simulink model "bicopter_control_comparison"  (R2023a)
settings: Solver=VariableStepAuto  StartTime=0.0  StopTime=20.0  RelTol=1e-3
libraries: fuzblock x4, simulink_extras x1
settings Model: Creator=KIIT  LastModifiedBy=tanay
settings OptimizationCC: ReuseModelBlockBuffer=off
settings DebuggingCC: UnconnectedInputMsg=warning  UnconnectedOutputMsg=warning  UnconnectedLineMsg=warning
settings ModelReferenceCC: EnableRefExpFcnMdlSchedulingChecks=on
settings RTWCC: DLArmComputeVersion=19.05

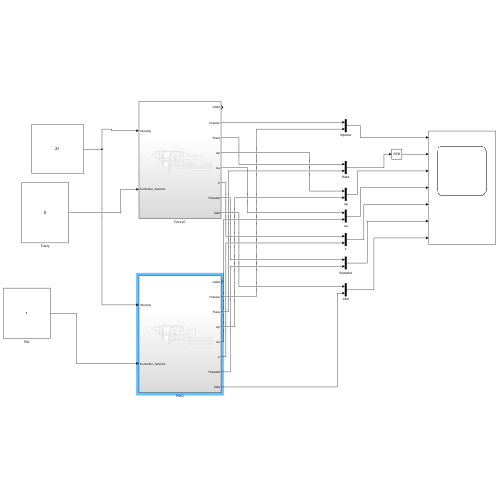
[thumbnail: Simulink's stored preview of the top-level diagram]
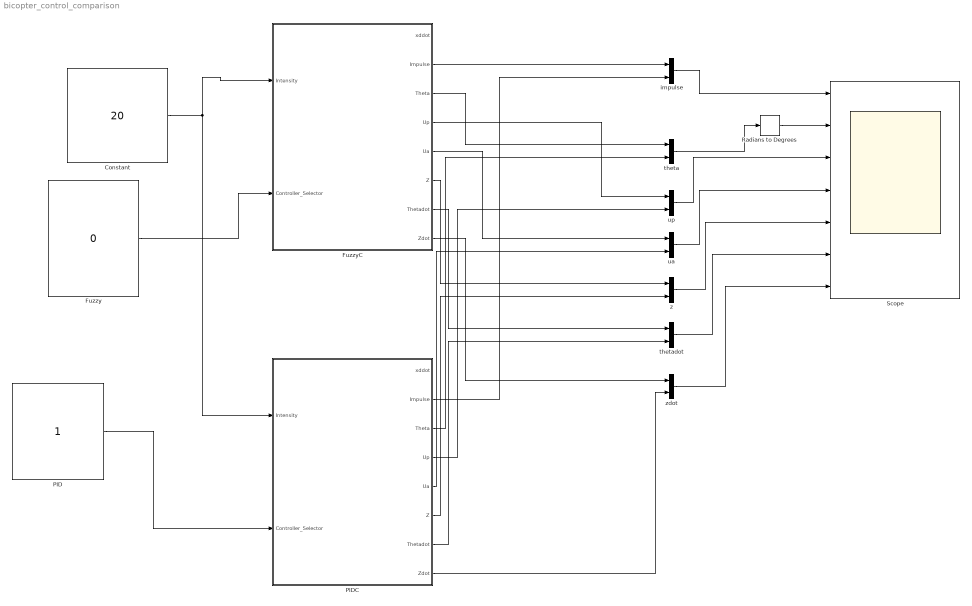
== system bicopter_control_comparison ==
  Constant : Constant  Value=20
  Fuzzy : Constant  Value=0
  FuzzyC : Subsystem
  PID : Constant
  PIDC : Subsystem
  Radians to Degrees : simulink_extras/Transformations/Radians to Degrees
  Scope : Scope  NumInputPorts=7
  impulse : Mux  Inputs=2
  theta : Mux  Inputs=2
  thetadot : Mux  Inputs=2
  ua : Mux  Inputs=2
  up : Mux  Inputs=2
  z : Mux  Inputs=2
  zdot : Mux  Inputs=2
  wires:
  Constant/1 -> FuzzyC/1(Intensity), PIDC/1(Intensity)
  PID/1 -> PIDC/2(Controller_Selector)
  Fuzzy/1 -> FuzzyC/2(Controller_Selector)
  FuzzyC/2(Impulse) -> impulse/1
  PIDC/2(Impulse) -> impulse/2
  FuzzyC/3(Theta) -> theta/1
  PIDC/3(Theta) -> theta/2
  FuzzyC/4(Up) -> up/1
  PIDC/4(Up) -> up/2
  FuzzyC/5(Ua) -> ua/1
  FuzzyC/6(Z) -> z/1
  FuzzyC/7(Thetadot) -> thetadot/1
  FuzzyC/8(Zdot) -> zdot/1
  PIDC/5(Ua) -> ua/2
  PIDC/6(Z) -> z/2
  PIDC/7(Thetadot) -> thetadot/2
  PIDC/8(Zdot) -> zdot/2
  impulse/1 -> Scope/1
  up/1 -> Scope/3
  ua/1 -> Scope/4
  z/1 -> Scope/5
  thetadot/1 -> Scope/6
  zdot/1 -> Scope/7
  theta/1 -> Radians to Degrees/1
  Radians to Degrees/1 -> Scope/2

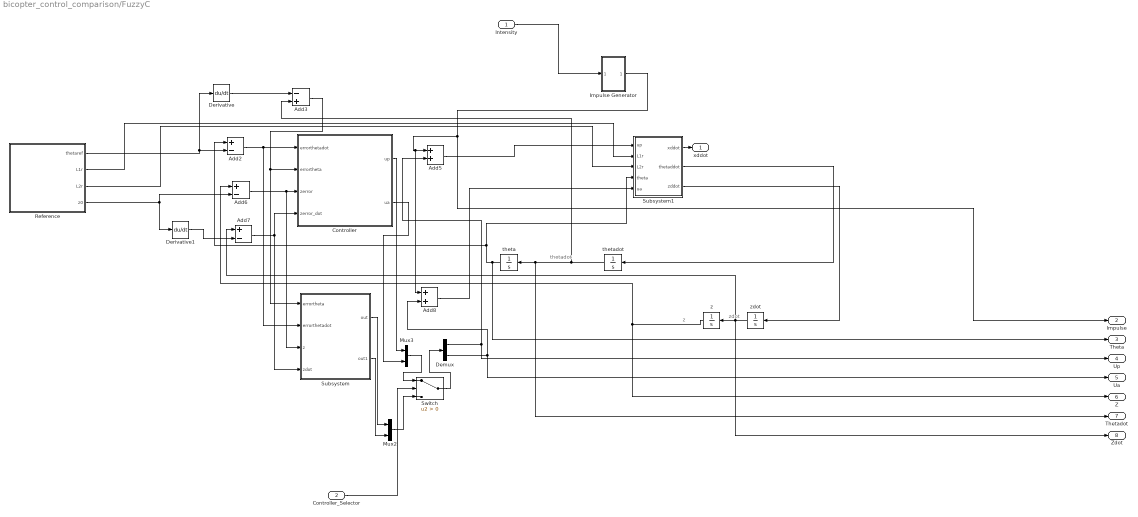
== system bicopter_control_comparison/FuzzyC ==
  note: z
  note: zdot
  note: thetadot
  Intensity : Inport
  Controller_Selector : Inport  Port=2
  Add2 : Sum  Inputs=+-
  Add3 : Sum  Inputs=-+
  Add5 : Sum
  Add6 : Sum  Inputs=+-
  Add7 : Sum  Inputs=+-
  Add8 : Sum
  Controller : Subsystem
  Demux : Demux  Outputs=2
  Derivative : Derivative
  Derivative1 : Derivative
  Impulse Generator : Subsystem
  Mux2 : Mux  Inputs=2
  Mux3 : Mux  Inputs=2
  Reference : MATLAB Function  TreatAsAtomicUnit=on
  Subsystem : Subsystem
  Subsystem1 : Subsystem
  Switch : Switch  Criteria=u2 > Threshold  SaturateOnIntegerOverflow=off  InputSameDT=off
  theta : Integrator  WrapState=on
  thetadot : Integrator
  z : Integrator
  zdot : Integrator
  xddot : Outport
  Impulse : Outport  Port=2
  Theta : Outport  Port=3
  Up : Outport  Port=4
  Ua : Outport  Port=5
  Z : Outport  Port=6
  Thetadot : Outport  Port=7
  Zdot : Outport  Port=8
  wires:
  Add7/1 -> Subsystem/4(zdot), Controller/4(zerror_dot)
  Reference/4(z0) -> Derivative1/1, Add6/2
  Intensity/1 -> Impulse Generator/1(Intensity)
  Subsystem/2(out1) -> Mux2/2
  zdot/1 -> Zdot/1, Add7/1, z/1
  Reference/1(thetaref) -> Add2/2, Derivative/1
  Add6/1 -> Subsystem/3(z), Controller/3(zerror)
  Controller/2(ua) -> Mux3/2
  z/1 -> Z/1, Add6/1
  Add2/1 -> Subsystem/2(errorthetadot), Controller/1(errorthetadot)
  Add3/1 -> Subsystem/1(errortheta), Controller/2(errortheta)
  Add5/1 -> Subsystem1/1(up)
  Subsystem/1(out) -> Mux2/1
  theta/1 -> Theta/1, Subsystem1/4(theta), Add2/1
  Demux/1 -> Add5/2, Up/1
  Derivative/1 -> Add3/1
  Controller/1(up) -> Mux3/1
  Impulse Generator/1(Out1) -> Impulse/1, Add8/1, Add5/1
  Reference/2(L1r) -> Subsystem1/2(L1r)
  Derivative1/1 -> Add7/2
  Subsystem1/3(zddot) -> zdot/1
  Subsystem1/1(xddot) -> xddot/1
  thetadot/1 -> Add3/2, Thetadot/1, theta/1
  Demux/2 -> Add8/2, Ua/1
  Switch/1 -> Demux/1
  Mux2/1 -> Switch/3
  Add8/1 -> Subsystem1/5(ua)
  Mux3/1 -> Switch/1
  Subsystem1/2(thetaddot) -> thetadot/1
  Controller_Selector/1 -> Switch/2
  Reference/3(L2r) -> Subsystem1/3(L2r)

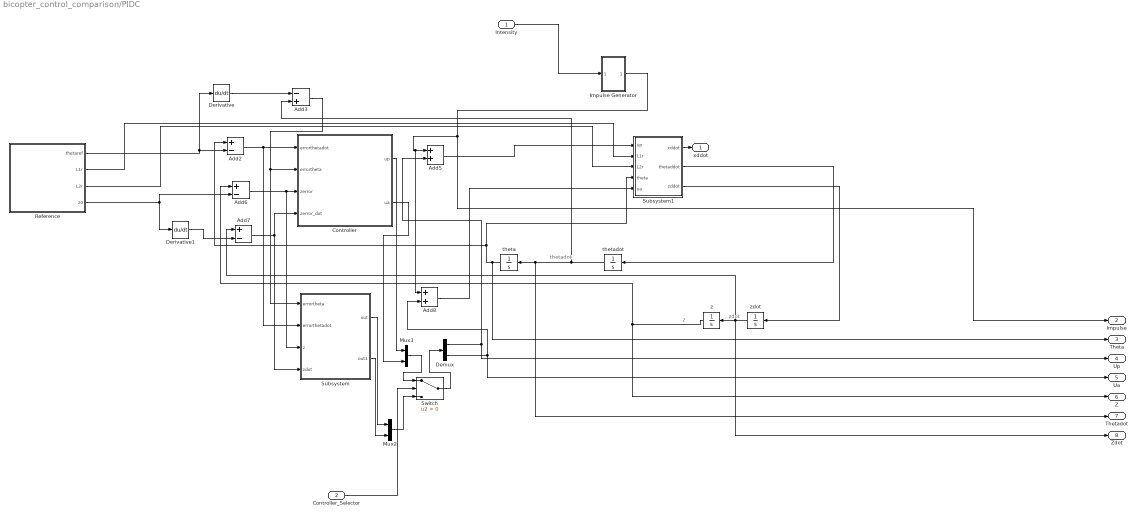
== system bicopter_control_comparison/PIDC ==
  note: z
  note: zdot
  note: thetadot
  Intensity : Inport
  Controller_Selector : Inport  Port=2
  Add2 : Sum  Inputs=+-
  Add3 : Sum  Inputs=-+
  Add5 : Sum
  Add6 : Sum  Inputs=+-
  Add7 : Sum  Inputs=+-
  Add8 : Sum
  Controller : Subsystem
  Demux : Demux  Outputs=2
  Derivative : Derivative
  Derivative1 : Derivative
  Impulse Generator : Subsystem
  Mux2 : Mux  Inputs=2
  Mux3 : Mux  Inputs=2
  Reference : MATLAB Function  TreatAsAtomicUnit=on
  Subsystem : Subsystem
  Subsystem1 : Subsystem
  Switch : Switch  Criteria=u2 > Threshold  SaturateOnIntegerOverflow=off  InputSameDT=off
  theta : Integrator  WrapState=on
  thetadot : Integrator
  z : Integrator
  zdot : Integrator
  xddot : Outport
  Impulse : Outport  Port=2
  Theta : Outport  Port=3
  Up : Outport  Port=4
  Ua : Outport  Port=5
  Z : Outport  Port=6
  Thetadot : Outport  Port=7
  Zdot : Outport  Port=8
  wires:
  Add7/1 -> Subsystem/4(zdot), Controller/4(zerror_dot)
  Reference/4(z0) -> Derivative1/1, Add6/2
  Intensity/1 -> Impulse Generator/1(Intensity)
  Subsystem/2(out1) -> Mux2/2
  zdot/1 -> Zdot/1, Add7/1, z/1
  Reference/1(thetaref) -> Add2/2, Derivative/1
  Add6/1 -> Subsystem/3(z), Controller/3(zerror)
  Controller/2(ua) -> Mux3/2
  z/1 -> Z/1, Add6/1
  Add2/1 -> Subsystem/2(errorthetadot), Controller/1(errorthetadot)
  Add3/1 -> Subsystem/1(errortheta), Controller/2(errortheta)
  Add5/1 -> Subsystem1/1(up)
  Subsystem/1(out) -> Mux2/1
  theta/1 -> Theta/1, Subsystem1/4(theta), Add2/1
  Demux/1 -> Add5/2, Up/1
  Derivative/1 -> Add3/1
  Controller/1(up) -> Mux3/1
  Impulse Generator/1(Out1) -> Impulse/1, Add8/1, Add5/1
  Reference/2(L1r) -> Subsystem1/2(L1r)
  Derivative1/1 -> Add7/2
  Subsystem1/3(zddot) -> zdot/1
  Subsystem1/1(xddot) -> xddot/1
  thetadot/1 -> Add3/2, Thetadot/1, theta/1
  Demux/2 -> Add8/2, Ua/1
  Switch/1 -> Demux/1
  Mux2/1 -> Switch/3
  Add8/1 -> Subsystem1/5(ua)
  Mux3/1 -> Switch/1
  Subsystem1/2(thetaddot) -> thetadot/1
  Controller_Selector/1 -> Switch/2
  Reference/3(L2r) -> Subsystem1/3(L2r)

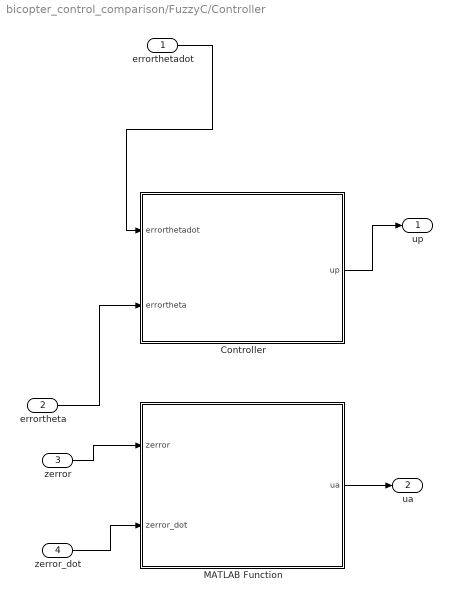
== system bicopter_control_comparison/FuzzyC/Controller ==
  errorthetadot : Inport
  errortheta : Inport  Port=2
  zerror : Inport  Port=3
  zerror_dot : Inport  Port=4
  Controller : MATLAB Function  TreatAsAtomicUnit=on
  MATLAB Function : MATLAB Function  TreatAsAtomicUnit=on
  up : Outport
  ua : Outport  Port=2
  wires:
  errortheta/1 -> Controller/2(errortheta)
  MATLAB Function/1(ua) -> ua/1
  errorthetadot/1 -> Controller/1(errorthetadot)
  zerror/1 -> MATLAB Function/1(zerror)
  Controller/1(up) -> up/1
  zerror_dot/1 -> MATLAB Function/2(zerror_dot)

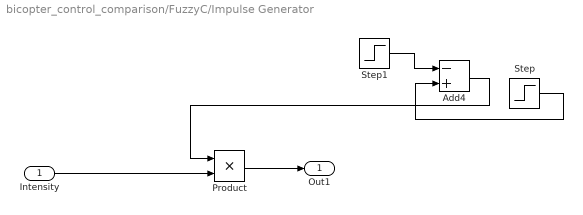
== system bicopter_control_comparison/FuzzyC/Impulse Generator ==
  Intensity : Inport
  Add4 : Sum  Inputs=-+
  Product : Product
  Step : Step  SampleTime=0
  Step1 : Step  Time=2  SampleTime=0
  Out1 : Outport
  wires:
  Step1/1 -> Add4/1
  Step/1 -> Add4/2
  Add4/1 -> Product/1
  Product/1 -> Out1/1
  Intensity/1 -> Product/2

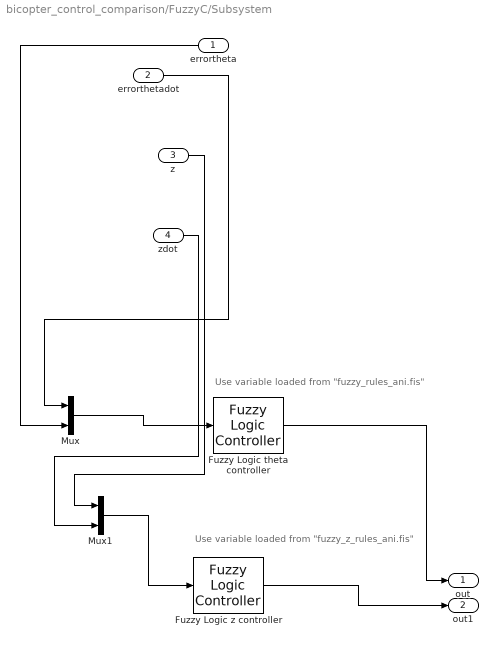
== system bicopter_control_comparison/FuzzyC/Subsystem ==
  note: Use variable loaded from "fuzzy_rules_ani.fis"
  note: Use variable loaded from "fuzzy_z_rules_ani.fis"
  errortheta : Inport
  errorthetadot : Inport  Port=2
  z : Inport  Port=3
  zdot : Inport  Port=4
  Fuzzy Logic theta controller : fuzblock/Fuzzy Logic  Controller  FIS=fuzzy_rules_ani  OutputSampleNumber=101  DataType=double  FuzzifiedInputs=off  RuleFiringStrengths=off  RuleOutputs=off  AggregatedOutputs=off  SimulateUsing=Interpreted execution  OutOfRangeInputValueMessage=warning  NoRuleFiredMessage=warning  EmptyOutputFuzzySetMessage=warning
  Fuzzy Logic z controller : fuzblock/Fuzzy Logic  Controller  FIS=fuzzy_z_rules_ani  OutputSampleNumber=101  DataType=double  FuzzifiedInputs=off  RuleFiringStrengths=off  RuleOutputs=off  AggregatedOutputs=off  SimulateUsing=Interpreted execution  OutOfRangeInputValueMessage=warning  NoRuleFiredMessage=warning  EmptyOutputFuzzySetMessage=warning
  Mux : Mux  Inputs=2
  Mux1 : Mux  Inputs=2
  out : Outport
  out1 : Outport  Port=2
  wires:
  Mux1/1 -> Fuzzy Logic z controller/1
  z/1 -> Mux1/1
  Mux/1 -> Fuzzy Logic theta controller/1
  errorthetadot/1 -> Mux/1
  Fuzzy Logic z controller/1 -> out1/1
  zdot/1 -> Mux1/2
  Fuzzy Logic theta controller/1 -> out/1
  errortheta/1 -> Mux/2

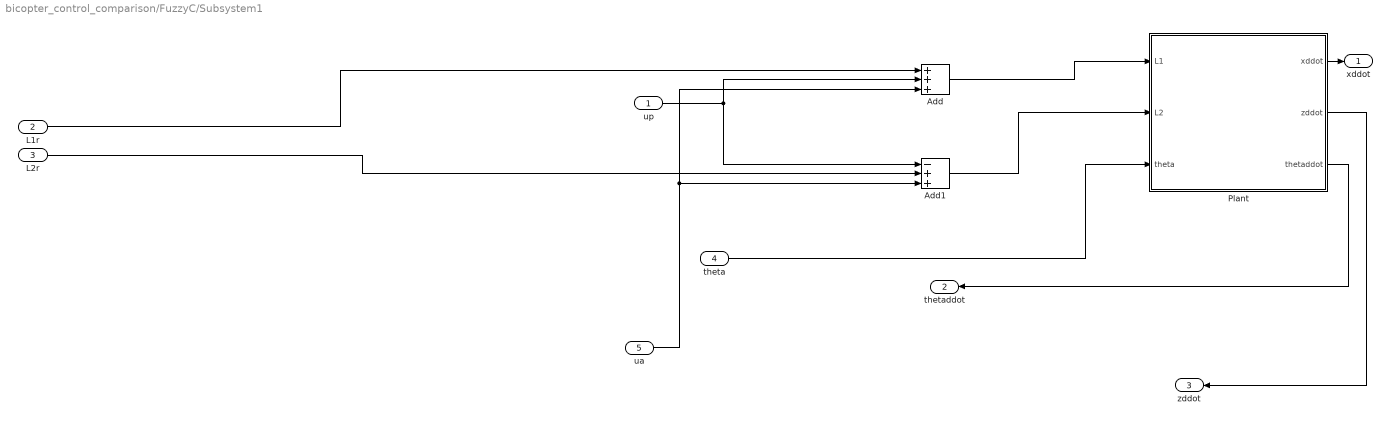
== system bicopter_control_comparison/FuzzyC/Subsystem1 ==
  up : Inport
  L1r : Inport  Port=2
  L2r : Inport  Port=3
  theta : Inport  Port=4
  ua : Inport  Port=5
  Add : Sum  Inputs=+++
  Add1 : Sum  Inputs=-++
  Plant : MATLAB Function  TreatAsAtomicUnit=on
  xddot : Outport
  thetaddot : Outport  Port=2
  zddot : Outport  Port=3
  wires:
  up/1 -> Add/2, Add1/1
  ua/1 -> Add/3, Add1/3
  L1r/1 -> Add/1
  Add1/1 -> Plant/2(L2)
  Plant/1(xddot) -> xddot/1
  Add/1 -> Plant/1(L1)
  L2r/1 -> Add1/2
  theta/1 -> Plant/3(theta)
  Plant/3(thetaddot) -> thetaddot/1
  Plant/2(zddot) -> zddot/1

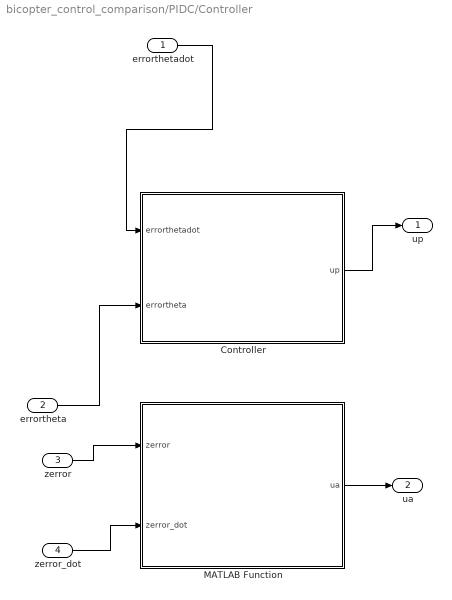
== system bicopter_control_comparison/PIDC/Controller ==
  errorthetadot : Inport
  errortheta : Inport  Port=2
  zerror : Inport  Port=3
  zerror_dot : Inport  Port=4
  Controller : MATLAB Function  TreatAsAtomicUnit=on
  MATLAB Function : MATLAB Function  TreatAsAtomicUnit=on
  up : Outport
  ua : Outport  Port=2
  wires:
  errortheta/1 -> Controller/2(errortheta)
  MATLAB Function/1(ua) -> ua/1
  errorthetadot/1 -> Controller/1(errorthetadot)
  zerror/1 -> MATLAB Function/1(zerror)
  Controller/1(up) -> up/1
  zerror_dot/1 -> MATLAB Function/2(zerror_dot)

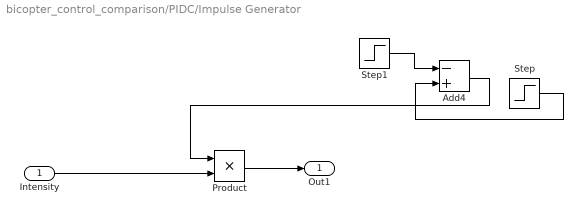
== system bicopter_control_comparison/PIDC/Impulse Generator ==
  Intensity : Inport
  Add4 : Sum  Inputs=-+
  Product : Product
  Step : Step  SampleTime=0
  Step1 : Step  Time=2  SampleTime=0
  Out1 : Outport
  wires:
  Step1/1 -> Add4/1
  Step/1 -> Add4/2
  Add4/1 -> Product/1
  Product/1 -> Out1/1
  Intensity/1 -> Product/2

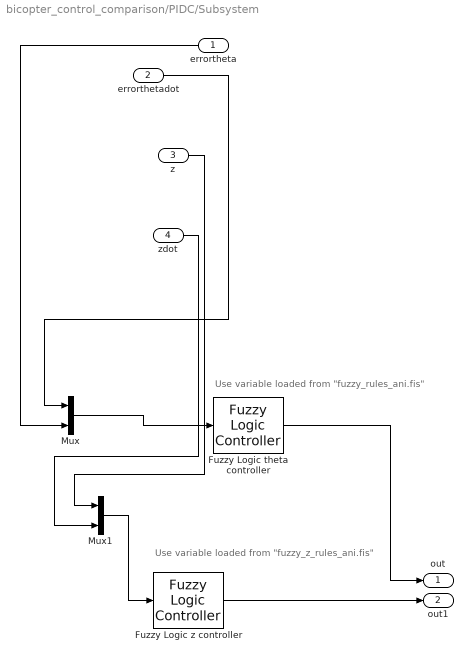
== system bicopter_control_comparison/PIDC/Subsystem ==
  note: Use variable loaded from "fuzzy_rules_ani.fis"
  note: Use variable loaded from "fuzzy_z_rules_ani.fis"
  errortheta : Inport
  errorthetadot : Inport  Port=2
  z : Inport  Port=3
  zdot : Inport  Port=4
  Fuzzy Logic theta controller : fuzblock/Fuzzy Logic  Controller  FIS=fuzzy_rules_ani  OutputSampleNumber=101  DataType=double  FuzzifiedInputs=off  RuleFiringStrengths=off  RuleOutputs=off  AggregatedOutputs=off  SimulateUsing=Interpreted execution  OutOfRangeInputValueMessage=warning  NoRuleFiredMessage=warning  EmptyOutputFuzzySetMessage=warning
  Fuzzy Logic z controller : fuzblock/Fuzzy Logic  Controller  FIS=fuzzy_z_rules_ani  OutputSampleNumber=101  DataType=double  FuzzifiedInputs=off  RuleFiringStrengths=off  RuleOutputs=off  AggregatedOutputs=off  SimulateUsing=Interpreted execution  OutOfRangeInputValueMessage=warning  NoRuleFiredMessage=warning  EmptyOutputFuzzySetMessage=warning
  Mux : Mux  Inputs=2
  Mux1 : Mux  Inputs=2
  out : Outport
  out1 : Outport  Port=2
  wires:
  Mux1/1 -> Fuzzy Logic z controller/1
  z/1 -> Mux1/1
  Mux/1 -> Fuzzy Logic theta controller/1
  errorthetadot/1 -> Mux/1
  Fuzzy Logic z controller/1 -> out1/1
  zdot/1 -> Mux1/2
  Fuzzy Logic theta controller/1 -> out/1
  errortheta/1 -> Mux/2

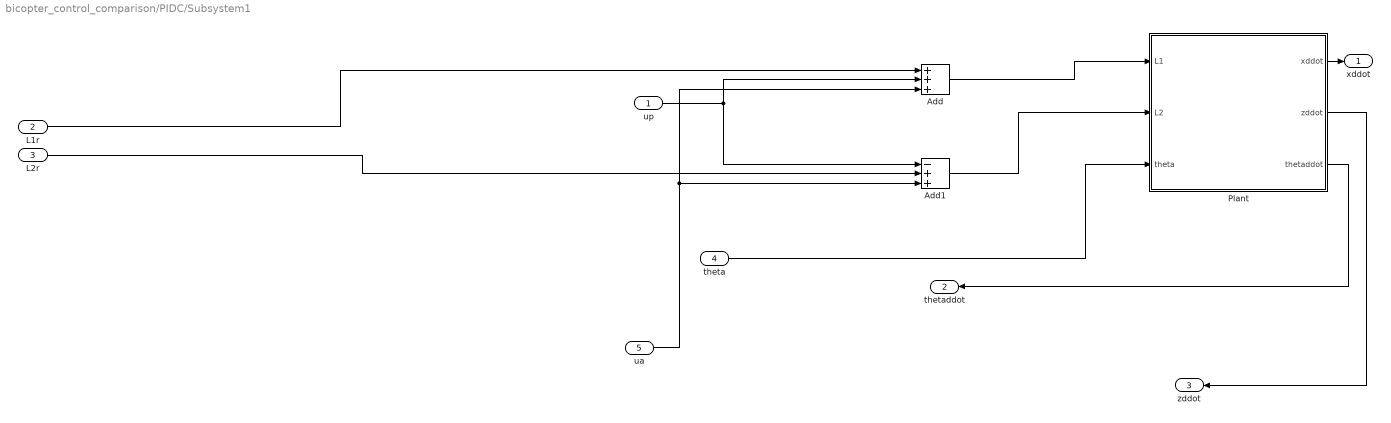
== system bicopter_control_comparison/PIDC/Subsystem1 ==
  up : Inport
  L1r : Inport  Port=2
  L2r : Inport  Port=3
  theta : Inport  Port=4
  ua : Inport  Port=5
  Add : Sum  Inputs=+++
  Add1 : Sum  Inputs=-++
  Plant : MATLAB Function  TreatAsAtomicUnit=on
  xddot : Outport
  thetaddot : Outport  Port=2
  zddot : Outport  Port=3
  wires:
  up/1 -> Add/2, Add1/1
  ua/1 -> Add/3, Add1/3
  L1r/1 -> Add/1
  Add1/1 -> Plant/2(L2)
  Plant/1(xddot) -> xddot/1
  Add/1 -> Plant/1(L1)
  L2r/1 -> Add1/2
  theta/1 -> Plant/3(theta)
  Plant/3(thetaddot) -> thetaddot/1
  Plant/2(zddot) -> zddot/1

== matlab function bicopter_control_comparison/FuzzyC/Subsystem1/Plant ==
  data: L1 input; xddot output; L2 input; theta input; zddot output; thetaddot output
function [xddot, zddot, thetaddot] = fcn(L1, L2, theta)
m = 2;
Iy = 0.2;
g = 9.8;
d = 0.2;
k1 = 24;
k2 = 7;
o1 = -(1/m)*(L1+L2)*sin(theta);
o2 = -(1/m)*(m*g - (L1+L2)*cos(theta));
o3 =(1/Iy)*d*(L1-L2);
xddot = o1;
zddot = o2;
thetaddot = o3;

== matlab function bicopter_control_comparison/FuzzyC/Controller/Controller ==
  data: errorthetadot input; up output; errortheta input
function up  = fcn(errorthetadot, errortheta)
m = 2;
Iy = 0.2;
g = 9.8;
d = 0.2;
k1 = 24;
k2 = 7;
up1 = (Iy/(2*d))*((1+k1)*errortheta + k2*errorthetadot);
up = -up1;

== matlab function bicopter_control_comparison/FuzzyC/Reference ==
  data: thetaref output; L1r output; L2r output; z0 output
function [thetaref, L1r, L2r, z0] = fcn()
m = 2;
Iy = 0.2;
g = 9.8;
d = 0.2;
k1 = 24;
k2 = 7;
u = [0, m*g/2, m*g/2];
thetaref = 0;
L1r = m*g/2;
L2r = m*g/2;
z0 = 0;

== matlab function bicopter_control_comparison/FuzzyC/Controller/MATLAB Function ==
  data: zerror input; ua output; zerror_dot input
function ua = fcn(zerror,zerror_dot)
m = 2;
g = 9.8;
d = 0.2;
k3 = 3;
k4 = 3;
ubar = m*((1+k3)*zerror+k4*zerror_dot);
ua = ubar/2.0;

== matlab function bicopter_control_comparison/PIDC/Controller/Controller ==
  data: errorthetadot input; up output; errortheta input
function up  = fcn(errorthetadot, errortheta)
m = 2;
Iy = 0.2;
g = 9.8;
d = 0.2;
k1 = 24;
k2 = 7;
up1 = (Iy/(2*d))*((1+k1)*errortheta + k2*errorthetadot);
up = -up1;

== matlab function bicopter_control_comparison/PIDC/Controller/MATLAB Function ==
  data: zerror input; ua output; zerror_dot input
function ua = fcn(zerror,zerror_dot)
m = 2;
g = 9.8;
d = 0.2;
k3 = 3;
k4 = 3;
ubar = m*((1+k3)*zerror+k4*zerror_dot);
ua = -ubar/2.0;

== matlab function bicopter_control_comparison/PIDC/Reference ==
  data: thetaref output; L1r output; L2r output; z0 output
function [thetaref, L1r, L2r, z0] = fcn()
m = 2;
Iy = 0.2;
g = 9.8;
d = 0.2;
k1 = 24;
k2 = 7;
u = [0, m*g/2, m*g/2];
thetaref = 0;
L1r = m*g/2;
L2r = m*g/2;
z0 = 0;

== matlab function bicopter_control_comparison/PIDC/Subsystem1/Plant ==
  data: L1 input; xddot output; L2 input; theta input; zddot output; thetaddot output
function [xddot, zddot, thetaddot] = fcn(L1, L2, theta)
m = 2;
Iy = 0.2;
g = 9.8;
d = 0.2;
k1 = 24;
k2 = 7;
o1 = -(1/m)*(L1+L2)*sin(theta);
o2 = -(1/m)*(m*g - (L1+L2)*cos(theta));
o3 =(1/Iy)*d*(L1-L2);
xddot = o1;
zddot = o2;
thetaddot = o3;
